simulink model "single_phase_gridonnected_ inverter_noPV_full"  (R2020b)
settings: Solver=FixedStepDiscrete  StartTime=0.0  StopTime=2  FixedStep=5e-7  MaxStep=1e-6  RelTol=1e-3
libraries: powerlib x53, simulink x4, pid_lib x2, discretizing x2
settings Model: SimulationMode=accelerator  Creator=zhaoy  LastModifiedBy=gc45
settings DataIOCC: ReturnWorkspaceOutputs=off
settings OptimizationCC: LifeSpan=inf
settings DebuggingCC: ArithmeticOperatorsInVariantConditions=warning
settings SFSimCC: SimUseLocalCustomCode=off  CustomCodeUndefinedFunction=UseInterfaceOnly
settings RTWCC: RTWUseLocalCustomCode=off
settings CodeAppCC: StateflowObjectComments=on
settings SimscapeCC: SimscapeNormalizeSystem=off

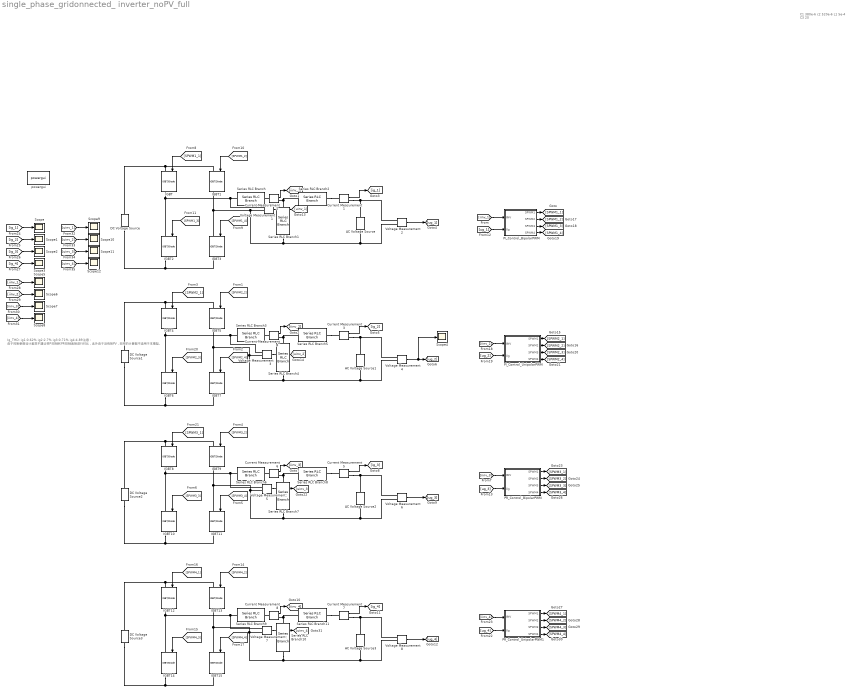
== system single_phase_gridonnected_ inverter_noPV_full ==
  note: Ig_THD:
      | ig1:0.62%
      | ig2:2.7%
      | ig3:0.71%
      | ig4:4.89%
      | 注意：
      | 由于控制参数设计差异不建议将PI控制和PR控制直接进行对比，此外由于没有接PV，效率的计算暂不适用于本模型。
  note: C1 380e-6
      | c2 520e-6
      | L1 5e-4
      | C3 20
  AC Voltage Source{,1..3} (4 alike) : powerlib/Electrical Sources/AC Voltage Source  Amplitude=311  Phase=0  Frequency=50  SampleTime=0  Measurements=None  BusType=swing  Pref=10e3  Qref=0  Qmin=-inf  Qmax=+inf
  Current Measurement{1..8} (8 alike) : powerlib/Measurements/Current Measurement  PhasorSimulation=off  OutputType=Complex  PSBequivalent=0
  DC Voltage Source{,1..3} (4 alike) : powerlib/Electrical Sources/DC Voltage Source  Amplitude=400  Measurements=None
  IGBT{,1..15} (16 alike) : powerlib/Power Electronics/IGBT//Diode  Ron=1e-3  Rs=1e5  Cs=inf  Measurements=on
  PI_Control_BipolarPWM : Subsystem
  PI_Control_UnipolarPWM : Subsystem
  PR_Control_BipolarPWM : Subsystem
  PR_Control_UnipolarPWM1 : Subsystem
  Scope{,1..12} (13 alike) : Scope
  Series RLC Branch : powerlib/Elements/Series RLC Branch  LConnTagsString=__new0  RConnTagsString=__new0  BranchType=L  Resistance=0.01  Inductance=4.08e-3  SetiL0=off  InitialCurrent=0  Capacitance=1e-6  Setx0=off  InitialVoltage=0  Measurements=None
  Series RLC Branch{1,4,7,10} (4 alike) : powerlib/Elements/Series RLC Branch  LConnTagsString=__new0  RConnTagsString=__new0  BranchType=C  Resistance=0.01  Inductance=20e-3  SetiL0=off  InitialCurrent=0  Capacitance=6e-6  Setx0=off  InitialVoltage=0  Measurements=None
  Series RLC Branch{2,5,8,11} (4 alike) : powerlib/Elements/Series RLC Branch  LConnTagsString=__new0  RConnTagsString=__new0  BranchType=L  Resistance=0.01  Inductance=4.35e-3  SetiL0=off  InitialCurrent=0  Capacitance=1e-6  Setx0=off  InitialVoltage=0  Measurements=None
  Series RLC Branch3 : powerlib/Elements/Series RLC Branch  LConnTagsString=__new0  RConnTagsString=__new0  BranchType=L  Resistance=0.01  Inductance=4.06e-3  SetiL0=off  InitialCurrent=0  Capacitance=1e-6  Setx0=off  InitialVoltage=0  Measurements=None
  Series RLC Branch6 : powerlib/Elements/Series RLC Branch  LConnTagsString=__new0  RConnTagsString=__new0  BranchType=L  Resistance=0.01  Inductance=4.06e-3  SetiL0=off  InitialCurrent=0  Capacitance=1e-6  Setx0=off  InitialVoltage=0  Measurements=None
  Series RLC Branch9 : powerlib/Elements/Series RLC Branch  LConnTagsString=__new0  RConnTagsString=__new0  BranchType=L  Resistance=0.01  Inductance=4.06e-3  SetiL0=off  InitialCurrent=0  Capacitance=1e-6  Setx0=off  InitialVoltage=0  Measurements=None
  Voltage Measurement{1..8} (8 alike) : powerlib/Measurements/Voltage Measurement  PhasorSimulation=off  OutputType=Complex  PSBequivalent=0
  powergui : powerlib/powergui  Priority=1  SimulationMode=Discrete  SampleTime=1e-6  frequency=50  Iterations=50  frequencyindice=50  Pbase=100e6  ErrMax=1e-4  UnitsV=kV  UnitsW=MW  buscounter=0  FunctionMessages=off  echomessages=off  EnableUseOfTLC=off  CurrentSourceSwitches=off  DisableSnubberDevices=off  DisableRonSwitches=off  DisableVfSwitches=off  DisplayEquations=off  AutomaticDiscreteSolvers=off  SolverType=Tustin/Backward Euler (TBE)  Interpol=off  ExternalGateDelay=off  methode=off  Ts=10  x0status=blocks  SPID=off  SwTol=0  HookPort=off  NonlinearTolerance=1e-4  nMaxIteration=100  ContinueOnMaxIteration=off  RestoreLinks=warning  ResistiveCurrentMeasurement=off  Frange=[0:2:500]  Ylog=off  Xlog=on  ShowGrid=off  save=off  variable=ZData  structure=ig1  ZoomFFT=off  StartTime=1  cycles=40  DisplayStyle=2  fundamental=50  FreqAxis=on  MaxFrequency=10000  frequencyindicesteady=1  RmsSteady=2  display=off
  wires:
  Current Measurement1/1 -> [ig_1]
  Voltage Measurement2/1 -> [ug_1]
  [SPWM1_1] -> IGBT/1
  [SPWM1_4] -> IGBT3/1
  [SPWM1_2] -> IGBT1/1
  [SPWM1_3] -> IGBT2/1
  [iinv_1] -> PI_Control_BipolarPWM/1(IINV)
  [ug_1] -> PI_Control_BipolarPWM/2(Ug)
  Current Measurement2/1 -> [iinv_1]
  [SPWM2_3] -> IGBT6/1
  [SPWM2_2] -> IGBT5/1
  Current Measurement4/1 -> [iinv_2]
  [SPWM2_1] -> IGBT4/1
  Current Measurement3/1 -> [ig_2]
  Voltage Measurement4/1 -> Scope4/1, [ug_2]
  [SPWM2_4] -> IGBT7/1
  Current Measurement6/1 -> [iinv_3]
  Current Measurement5/1 -> [ig_3]
  Voltage Measurement6/1 -> [ug_3]
  [SPWM4_3] -> IGBT14/1
  [SPWM4_2] -> IGBT13/1
  Current Measurement8/1 -> [iinv_4]
  [SPWM4_1] -> IGBT12/1
  Current Measurement7/1 -> [ig_4]
  Voltage Measurement8/1 -> [ug_4]
  [SPWM4_4] -> IGBT15/1
  Voltage Measurement1/1 -> [uinv_1]
  PI_Control_BipolarPWM/1(SPWM1) -> [SPWM1_1]
  PI_Control_BipolarPWM/2(SPWM2) -> [SPWM1_2]
  PI_Control_BipolarPWM/4(SPWM4) -> [SPWM1_4]
  PI_Control_BipolarPWM/3(SPWM3) -> [SPWM1_3]
  Voltage Measurement3/1 -> [uinv_2]
  PI_Control_UnipolarPWM/1(SPWM1) -> [SPWM2_1]
  PI_Control_UnipolarPWM/2(SPWM2) -> [SPWM2_2]
  PI_Control_UnipolarPWM/3(SPWM3) -> [SPWM2_3]
  PI_Control_UnipolarPWM/4(SPWM4) -> [SPWM2_4]
  [iinv_2] -> PI_Control_UnipolarPWM/1(IINV)
  [ug_2] -> PI_Control_UnipolarPWM/2(Ug)
  [SPWM3_2] -> IGBT9/1
  [SPWM3_1] -> IGBT8/1
  [SPWM3_4] -> IGBT11/1
  [SPWM3_3] -> IGBT10/1
  Voltage Measurement5/1 -> [uinv_3]
  PR_Control_BipolarPWM/2(SPWM2) -> [SPWM3_2]
  PR_Control_BipolarPWM/4(SPWM4) -> [SPWM3_4]
  PR_Control_BipolarPWM/1(SPWM1) -> [SPWM3_1]
  [iinv_3] -> PR_Control_BipolarPWM/1(IINV)
  [ug_3] -> PR_Control_BipolarPWM/2(Ug)
  PR_Control_BipolarPWM/3(SPWM3) -> [SPWM3_3]
  [ug_4] -> PR_Control_UnipolarPWM1/2(Ug)
  [iinv_4] -> PR_Control_UnipolarPWM1/1(IINV)
  PR_Control_UnipolarPWM1/2(SPWM2) -> [SPWM4_2]
  PR_Control_UnipolarPWM1/3(SPWM3) -> [SPWM4_3]
  PR_Control_UnipolarPWM1/4(SPWM4) -> [SPWM4_4]
  PR_Control_UnipolarPWM1/1(SPWM1) -> [SPWM4_1]
  Voltage Measurement7/1 -> [uinv_4]
  [ig_1] -> Scope/1
  [ig_4] -> Scope3/1
  [ig_2] -> Scope1/1
  [ig_3] -> Scope2/1
  [iinv_1] -> Scope5/1
  [iinv_2] -> Scope6/1
  [iinv_3] -> Scope7/1
  [iinv_4] -> Scope8/1
  [uinv_1] -> Scope9/1
  [uinv_2] -> Scope10/1
  [uinv_3] -> Scope11/1
  [uinv_4] -> Scope12/1
  connections:
  IGBT2/LConn1 -- Voltage Measurement1/LConn1 -- Series RLC Branch/LConn1 -- IGBT/RConn1
  IGBT3/LConn1 -- Series RLC Branch1/RConn1 -- Voltage Measurement2/LConn2 -- AC Voltage Source/LConn1 -- Voltage Measurement1/LConn2 -- IGBT1/RConn1
  IGBT2/RConn1 -- DC Voltage Source/LConn1 -- IGBT3/RConn1
  Current Measurement1/RConn1 -- AC Voltage Source/RConn1 -- Voltage Measurement2/LConn1
  Series RLC Branch2/LConn1 -- Current Measurement2/RConn1 -- Series RLC Branch1/LConn1
  IGBT1/LConn1 -- DC Voltage Source/RConn1 -- IGBT/LConn1
  Series RLC Branch2/RConn1 -- Current Measurement1/LConn1
  Current Measurement2/LConn1 -- Series RLC Branch/RConn1
  Series RLC Branch4/LConn1 -- Series RLC Branch5/LConn1 -- Current Measurement4/RConn1
  Voltage Measurement4/LConn1 -- Current Measurement3/RConn1 -- AC Voltage Source1/RConn1
  AC Voltage Source1/LConn1 -- IGBT7/LConn1 -- IGBT5/RConn1 -- Voltage Measurement3/LConn2 -- Series RLC Branch4/RConn1 -- Voltage Measurement4/LConn2
  IGBT4/LConn1 -- IGBT5/LConn1 -- DC Voltage Source1/RConn1
  IGBT4/RConn1 -- IGBT6/LConn1 -- Voltage Measurement3/LConn1 -- Series RLC Branch3/LConn1
  IGBT7/RConn1 -- IGBT6/RConn1 -- DC Voltage Source1/LConn1
  Series RLC Branch5/RConn1 -- Current Measurement3/LConn1
  Current Measurement4/LConn1 -- Series RLC Branch3/RConn1
  Series RLC Branch7/LConn1 -- Series RLC Branch8/LConn1 -- Current Measurement6/RConn1
  Voltage Measurement6/LConn1 -- Current Measurement5/RConn1 -- AC Voltage Source2/RConn1
  AC Voltage Source2/LConn1 -- IGBT11/LConn1 -- IGBT9/RConn1 -- Voltage Measurement5/LConn2 -- Series RLC Branch7/RConn1 -- Voltage Measurement6/LConn2
  IGBT8/LConn1 -- IGBT9/LConn1 -- DC Voltage Source2/RConn1
  IGBT8/RConn1 -- IGBT10/LConn1 -- Voltage Measurement5/LConn1 -- Series RLC Branch6/LConn1
  IGBT11/RConn1 -- IGBT10/RConn1 -- DC Voltage Source2/LConn1
  Series RLC Branch8/RConn1 -- Current Measurement5/LConn1
  Current Measurement6/LConn1 -- Series RLC Branch6/RConn1
  Series RLC Branch10/LConn1 -- Series RLC Branch11/LConn1 -- Current Measurement8/RConn1
  Voltage Measurement8/LConn1 -- Current Measurement7/RConn1 -- AC Voltage Source3/RConn1
  AC Voltage Source3/LConn1 -- IGBT15/LConn1 -- IGBT13/RConn1 -- Voltage Measurement7/LConn2 -- Series RLC Branch10/RConn1 -- Voltage Measurement8/LConn2
  IGBT12/LConn1 -- IGBT13/LConn1 -- DC Voltage Source3/RConn1
  IGBT12/RConn1 -- IGBT14/LConn1 -- Voltage Measurement7/LConn1 -- Series RLC Branch9/LConn1
  IGBT15/RConn1 -- IGBT14/RConn1 -- DC Voltage Source3/LConn1
  Series RLC Branch11/RConn1 -- Current Measurement7/LConn1
  Current Measurement8/LConn1 -- Series RLC Branch9/RConn1

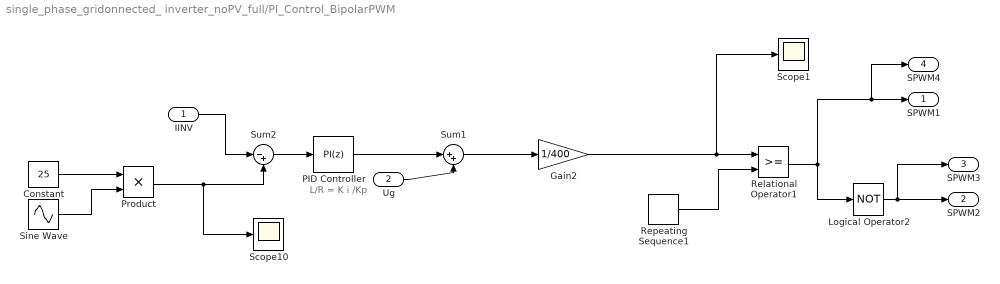
== system single_phase_gridonnected_ inverter_noPV_full/PI_Control_BipolarPWM ==
  note: L/R = K i /Kp
  IINV : Inport
  Ug : Inport  Port=2
  Constant : Constant  Value=25
  Gain2 : Gain  Gain=1/400
  Logical Operator2 : Logic  Operator=NOT  AllPortsSameDT=off  OutDataTypeStr=boolean
  PID Controller : pid_lib/PID Controller  Controller=PI  Form=Parallel  TimeDomain=Discrete-time  UseExternalTs=off  SampleTime=-1  IntegratorMethod=Forward Euler  FilterMethod=Forward Euler  ControllerParametersSource=internal  P=5  I=500  D=0  UseFilter=on  N=100  TunerSelectOption=Transfer Function Based (PID Tuner App)  InitialConditionSource=internal  InitialConditionForIntegrator=0  InitialConditionForFilter=0  DifferentiatorICPrevScaledInput=0  ExternalReset=none  TrackingMode=off  Kt=1  LimitOutput=off  SatLimitsSource=internal  UpperSaturationLimit=inf  LowerSaturationLimit=-inf  LinearizeAsGain=on  AntiWindupMode=none  Kb=1  POutMin=[]  POutMax=[]  IOutMin=[]  IOutMax=[]  DOutMin=[]  DOutMax=[]  NOutMin=[]  NOutMax=[]  SumOutMin=[]  SumOutMax=[]  SaturationOutMin=[]  SaturationOutMax=[]  PParamMin=[]  PParamMax=[]  IParamMin=[]  IParamMax=[]  DParamMin=[]  DParamMax=[]  NParamMin=[]  NParamMax=[]  KbParamMin=[]  KbParamMax=[]  KtParamMin=[]  KtParamMax=[]  KbOutMin=[]  KbOutMax=[]  KtOutMin=[]  KtOutMax=[]  IntegratorOutMin=[]  IntegratorOutMax=[]  FilterOutMin=[]  FilterOutMax=[]  SumI1OutMin=[]  SumI1OutMax=[]  SumI2OutMin=[]  SumI2OutMax=[]  SumI3OutMin=[]  SumI3OutMax=[]  SumI4OutMin=[]  SumI4OutMax=[]  SumDOutMin=[]  SumDOutMax=[]  DifferentiatorOutMin=[]  DifferentiatorOutMax=[]  FilterDiffOutCoefMin=[]  FilterDiffOutCoefMax=[]  ReciprocalOutMin=[]  ReciprocalOutMax=[]  SumDenOutMin=[]  SumDenOutMax=[]  SumNumOutMin=[]  SumNumOutMax=[]  DivideOutMin=[]  DivideOutMax=[]  UdiffTsProdOutMin=[]  UdiffTsProdOutMax=[]  NTsProdOutMin=[]  NTsProdOutMax=[]  UintegralTsProdOutMin=[]  UintegralTsProdOutMax=[]  UngainTsProdOutMin=[]  UngainTsProdOutMax=[]  IntegratorContinuousStateAttributes=''  IntegratorStateMustResolveToSignalObject=off  IntegratorRTWStateStorageClass=Auto  FilterContinuousStateAttributes=''  FilterStateMustResolveToSignalObject=off  FilterRTWStateStorageClass=Auto  ParallelPVariant=InternalParameters  IdealPVariant=Disabled  IVariant=InternalParameters  DVariant=Disabled  IntegratorVariant=Discrete  SatVariant=Disabled  AWVariant=Passthrough  PCopyVariant=Disabled  TRVariant=Disabled  FdbkBlocksVariant=Forward  IdealPFdbkVariant=Disabled  SatFdbkVariant=Disabled  DerivativeFilterVariant=Disabled  NVariant=Disabled  NCopyVariant=Disabled_SignalSpec  FilterICVariant=Disabled  IntegratorICVariant=InternalICs  ExternalResetVariant=Disabled  TRSumVariant=Passthrough  SumFdbkVariant=Disabled  SumVariant=Sum_PI  TsampFilterVariant=InternalTs  TsampNgainVariant=Passthrough  TsampIntegralVariant=Passthrough  ExternalSaturationOutDataTypeStr=Inherit: Same as second input
  Product : Product
  Relational Operator1 : RelationalOperator  OutDataTypeStr=boolean  RndMeth=Simplest
  Repeating Sequence1 : simulink/Sources/Repeating Sequence  rep_seq_t=[0 1/20000 1/10000]  rep_seq_y=[-1 1 -1]
  Scope1 : Scope
  Scope10 : Scope
  Sine Wave : Sin  Frequency=100*pi
  Sum1 : Sum  Inputs=|++
  Sum2 : Sum  Inputs=|-+
  SPWM1 : Outport
  SPWM2 : Outport  Port=2
  SPWM3 : Outport  Port=3
  SPWM4 : Outport  Port=4
  wires:
  Sum2/1 -> PID Controller/1
  Product/1 -> Scope10/1, Sum2/2
  IINV/1 -> Sum2/1
  Constant/1 -> Product/1
  Sine Wave/1 -> Product/2
  Ug/1 -> Sum1/2
  PID Controller/1 -> Sum1/1
  Sum1/1 -> Gain2/1
  Relational Operator1/1 -> SPWM4/1, SPWM1/1, Logical Operator2/1
  Gain2/1 -> Scope1/1, Relational Operator1/1
  Repeating Sequence1/1 -> Relational Operator1/2
  Logical Operator2/1 -> SPWM3/1, SPWM2/1

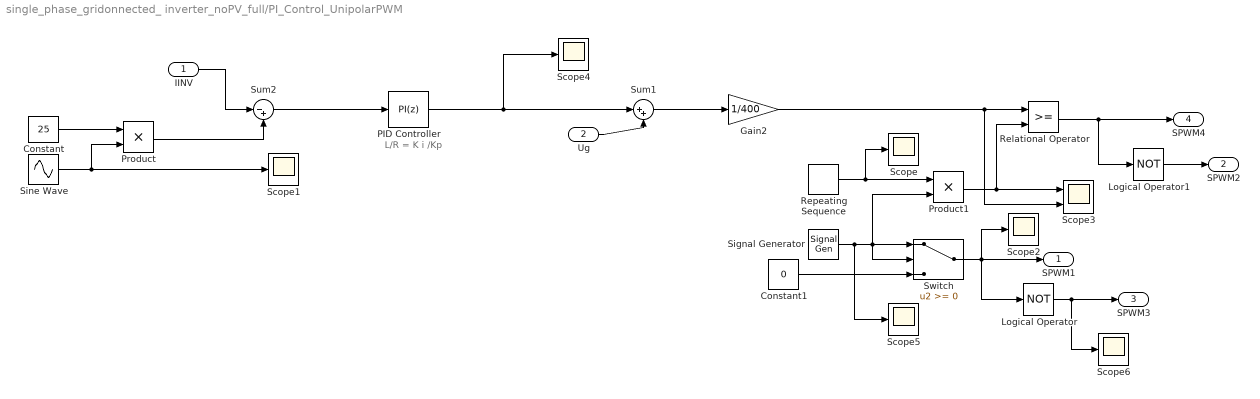
== system single_phase_gridonnected_ inverter_noPV_full/PI_Control_UnipolarPWM ==
  note: L/R = K i /Kp
  IINV : Inport
  Ug : Inport  Port=2
  Constant : Constant  Value=25
  Constant1 : Constant  Value=0
  Gain2 : Gain  Gain=1/400
  Logical Operator : Logic  Operator=NOT  AllPortsSameDT=off  OutDataTypeStr=boolean
  Logical Operator1 : Logic  Operator=NOT  AllPortsSameDT=off  OutDataTypeStr=boolean
  PID Controller : pid_lib/PID Controller  Controller=PI  Form=Parallel  TimeDomain=Discrete-time  UseExternalTs=off  SampleTime=-1  IntegratorMethod=Forward Euler  FilterMethod=Forward Euler  ControllerParametersSource=internal  P=5  I=500  D=0  UseFilter=on  N=100  TunerSelectOption=Transfer Function Based (PID Tuner App)  InitialConditionSource=internal  InitialConditionForIntegrator=0  InitialConditionForFilter=0  DifferentiatorICPrevScaledInput=0  ExternalReset=none  TrackingMode=off  Kt=1  LimitOutput=off  SatLimitsSource=internal  UpperSaturationLimit=inf  LowerSaturationLimit=-inf  LinearizeAsGain=on  AntiWindupMode=none  Kb=1  POutMin=[]  POutMax=[]  IOutMin=[]  IOutMax=[]  DOutMin=[]  DOutMax=[]  NOutMin=[]  NOutMax=[]  SumOutMin=[]  SumOutMax=[]  SaturationOutMin=[]  SaturationOutMax=[]  PParamMin=[]  PParamMax=[]  IParamMin=[]  IParamMax=[]  DParamMin=[]  DParamMax=[]  NParamMin=[]  NParamMax=[]  KbParamMin=[]  KbParamMax=[]  KtParamMin=[]  KtParamMax=[]  KbOutMin=[]  KbOutMax=[]  KtOutMin=[]  KtOutMax=[]  IntegratorOutMin=[]  IntegratorOutMax=[]  FilterOutMin=[]  FilterOutMax=[]  SumI1OutMin=[]  SumI1OutMax=[]  SumI2OutMin=[]  SumI2OutMax=[]  SumI3OutMin=[]  SumI3OutMax=[]  SumI4OutMin=[]  SumI4OutMax=[]  SumDOutMin=[]  SumDOutMax=[]  DifferentiatorOutMin=[]  DifferentiatorOutMax=[]  FilterDiffOutCoefMin=[]  FilterDiffOutCoefMax=[]  ReciprocalOutMin=[]  ReciprocalOutMax=[]  SumDenOutMin=[]  SumDenOutMax=[]  SumNumOutMin=[]  SumNumOutMax=[]  DivideOutMin=[]  DivideOutMax=[]  UdiffTsProdOutMin=[]  UdiffTsProdOutMax=[]  NTsProdOutMin=[]  NTsProdOutMax=[]  UintegralTsProdOutMin=[]  UintegralTsProdOutMax=[]  UngainTsProdOutMin=[]  UngainTsProdOutMax=[]  IntegratorContinuousStateAttributes=''  IntegratorStateMustResolveToSignalObject=off  IntegratorRTWStateStorageClass=Auto  FilterContinuousStateAttributes=''  FilterStateMustResolveToSignalObject=off  FilterRTWStateStorageClass=Auto  ParallelPVariant=InternalParameters  IdealPVariant=Disabled  IVariant=InternalParameters  DVariant=Disabled  IntegratorVariant=Discrete  SatVariant=Disabled  AWVariant=Passthrough  PCopyVariant=Disabled  TRVariant=Disabled  FdbkBlocksVariant=Forward  IdealPFdbkVariant=Disabled  SatFdbkVariant=Disabled  DerivativeFilterVariant=Disabled  NVariant=Disabled  NCopyVariant=Disabled_SignalSpec  FilterICVariant=Disabled  IntegratorICVariant=InternalICs  ExternalResetVariant=Disabled  TRSumVariant=Passthrough  SumFdbkVariant=Disabled  SumVariant=Sum_PI  TsampFilterVariant=InternalTs  TsampNgainVariant=Passthrough  TsampIntegralVariant=Passthrough  ExternalSaturationOutDataTypeStr=Inherit: Same as second input
  Product : Product
  Product1 : Product
  Relational Operator : RelationalOperator  OutDataTypeStr=boolean  RndMeth=Simplest
  Repeating Sequence : simulink/Sources/Repeating Sequence  rep_seq_t=[0 1/20000 1/10000]  rep_seq_y=[0 1 0]
  Scope{,1..2,4..6} (6 alike) : Scope
  Scope3 : Scope  NumInputPorts=2
  Signal Generator : SignalGenerator  WaveForm=square  Amplitude=-1  Frequency=50*2*pi  Units=rad/sec
  Sine Wave : Sin  Frequency=100*pi
  Sum1 : Sum  Inputs=|++
  Sum2 : Sum  Inputs=|-+
  Switch : Switch
  SPWM1 : Outport
  SPWM2 : Outport  Port=2
  SPWM3 : Outport  Port=3
  SPWM4 : Outport  Port=4
  wires:
  Sum2/1 -> PID Controller/1
  Product/1 -> Sum2/2
  IINV/1 -> Sum2/1
  Constant/1 -> Product/1
  Sine Wave/1 -> Scope1/1, Product/2
  Ug/1 -> Sum1/2
  Signal Generator/1 -> Scope5/1, Product1/2, Switch/2, Switch/1
  Repeating Sequence/1 -> Scope/1, Product1/1
  Product1/1 -> Relational Operator/2, Scope3/1
  Constant1/1 -> Switch/3
  Switch/1 -> SPWM1/1, Logical Operator/1, Scope2/1
  PID Controller/1 -> Scope4/1, Sum1/1
  Sum1/1 -> Gain2/1
  Gain2/1 -> Scope3/2, Relational Operator/1
  Relational Operator/1 -> Logical Operator1/1, SPWM4/1
  Logical Operator1/1 -> SPWM2/1
  Logical Operator/1 -> SPWM3/1, Scope6/1

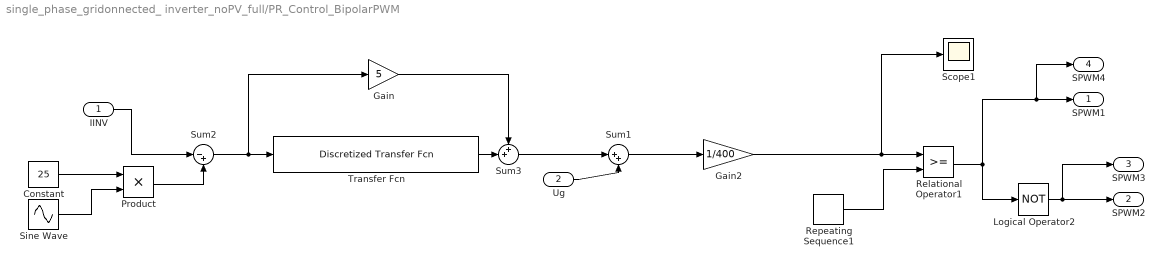
== system single_phase_gridonnected_ inverter_noPV_full/PR_Control_BipolarPWM ==
  IINV : Inport
  Ug : Inport  Port=2
  Constant : Constant  Value=25
  Gain : Gain  Gain=5
  Gain2 : Gain  Gain=1/400
  Logical Operator2 : Logic  Operator=NOT  AllPortsSameDT=off  OutDataTypeStr=boolean
  Product : Product
  Relational Operator1 : RelationalOperator  OutDataTypeStr=boolean  RndMeth=Simplest
  Repeating Sequence1 : simulink/Sources/Repeating Sequence  rep_seq_t=[0 1/20000 1/10000]  rep_seq_y=[-1 1 -1]
  Scope1 : Scope
  Sine Wave : Sin  Frequency=100*pi
  Sum1 : Sum  Inputs=|++
  Sum2 : Sum  Inputs=|-+
  Sum3 : Sum  Inputs=++|
  Transfer Fcn : discretizing/Discretized Transfer Fcn  Numerator=[2*400*2*pi 0]  Denominator=[1 2*2*pi 100*100*pi*pi]  AbsTol=auto  SampleTime=5e-7  method=zoh  Wc=1
      settings: SourceProductBaseCode=SL
  SPWM1 : Outport
  SPWM2 : Outport  Port=2
  SPWM3 : Outport  Port=3
  SPWM4 : Outport  Port=4
  wires:
  Sum2/1 -> Transfer Fcn/1, Gain/1
  Product/1 -> Sum2/2
  IINV/1 -> Sum2/1
  Constant/1 -> Product/1
  Sine Wave/1 -> Product/2
  Ug/1 -> Sum1/2
  Sum3/1 -> Sum1/1
  Sum1/1 -> Gain2/1
  Gain2/1 -> Scope1/1, Relational Operator1/1
  Relational Operator1/1 -> SPWM4/1, SPWM1/1, Logical Operator2/1
  Repeating Sequence1/1 -> Relational Operator1/2
  Logical Operator2/1 -> SPWM3/1, SPWM2/1
  Transfer Fcn/1 -> Sum3/2
  Gain/1 -> Sum3/1

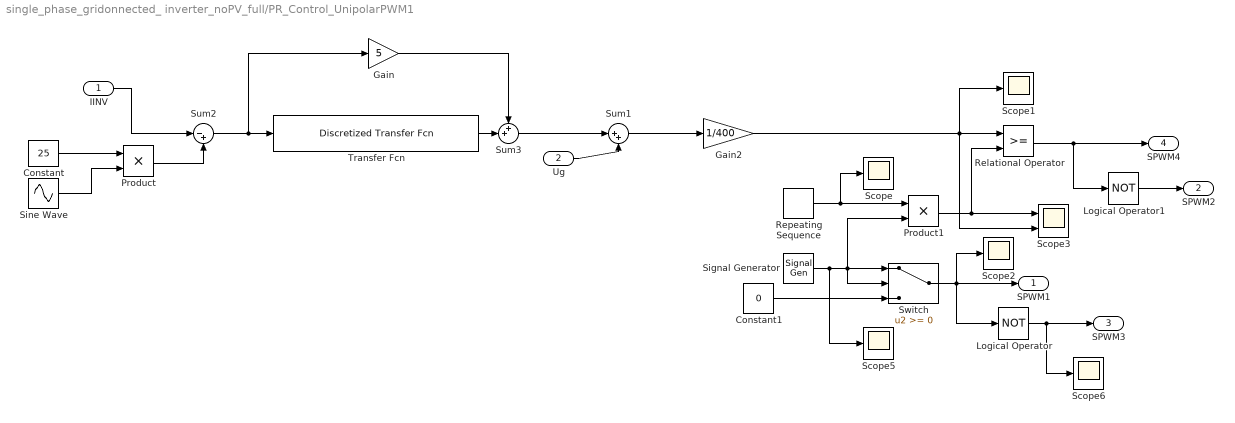
== system single_phase_gridonnected_ inverter_noPV_full/PR_Control_UnipolarPWM1 ==
  IINV : Inport
  Ug : Inport  Port=2
  Constant : Constant  Value=25
  Constant1 : Constant  Value=0
  Gain : Gain  Gain=5
  Gain2 : Gain  Gain=1/400
  Logical Operator : Logic  Operator=NOT  AllPortsSameDT=off  OutDataTypeStr=boolean
  Logical Operator1 : Logic  Operator=NOT  AllPortsSameDT=off  OutDataTypeStr=boolean
  Product : Product
  Product1 : Product
  Relational Operator : RelationalOperator  OutDataTypeStr=boolean  RndMeth=Simplest
  Repeating Sequence : simulink/Sources/Repeating Sequence  rep_seq_t=[0 1/20000 1/10000]  rep_seq_y=[0 1 0]
  Scope{,1..2,5..6} (5 alike) : Scope
  Scope3 : Scope  NumInputPorts=2
  Signal Generator : SignalGenerator  WaveForm=square  Amplitude=-1  Frequency=50*2*pi  Units=rad/sec
  Sine Wave : Sin  Frequency=100*pi
  Sum1 : Sum  Inputs=|++
  Sum2 : Sum  Inputs=|-+
  Sum3 : Sum  Inputs=++|
  Switch : Switch
  Transfer Fcn : discretizing/Discretized Transfer Fcn  Numerator=[2*400*2*pi 0]  Denominator=[1 2*2*pi 100*100*pi*pi]  AbsTol=auto  SampleTime=5e-7  method=zoh  Wc=1
      settings: SourceProductBaseCode=SL
  SPWM1 : Outport
  SPWM2 : Outport  Port=2
  SPWM3 : Outport  Port=3
  SPWM4 : Outport  Port=4
  wires:
  Sum2/1 -> Transfer Fcn/1, Gain/1
  Product/1 -> Sum2/2
  IINV/1 -> Sum2/1
  Constant/1 -> Product/1
  Sine Wave/1 -> Product/2
  Ug/1 -> Sum1/2
  Sum3/1 -> Sum1/1
  Sum1/1 -> Gain2/1
  Transfer Fcn/1 -> Sum3/2
  Gain/1 -> Sum3/1
  Gain2/1 -> Scope1/1, Scope3/2, Relational Operator/1
  Logical Operator1/1 -> SPWM2/1
  Repeating Sequence/1 -> Scope/1, Product1/1
  Relational Operator/1 -> Logical Operator1/1, SPWM4/1
  Logical Operator/1 -> SPWM3/1, Scope6/1
  Switch/1 -> SPWM1/1, Logical Operator/1, Scope2/1
  Constant1/1 -> Switch/3
  Signal Generator/1 -> Scope5/1, Product1/2, Switch/2, Switch/1
  Product1/1 -> Relational Operator/2, Scope3/1
